simulink model "Nexonar_Test"  (R2018b)
settings: Solver=FixedStepDiscrete  StartTime=0.0  StopTime=7.5  RelTol=1e-3  EnableMultiTasking=on
(part 1 of 2)
settings Model: ExtModeTrigDuration=8  Creator=User  LastModifiedBy=hengw
settings DataIOCC: LimitDataPoints=on  SaveFormat=Array  SaveOutput=off  SaveTime=off
settings OptimizationCC: DefaultUnderspecifiedDataType=single  ExpressionDepthLimit=2147483647  LifeSpan=1  MaxStackSize=512
settings DebuggingCC: UnderspecifiedInitializationDetection=Classic  MergeDetectMultiDrivingBlocksExec=none  SolverPrmCheckMsg=warning  StateNameClashWarn=warning  SFUnexpectedBacktrackingDiag=warning  SFNoUnconditionalDefaultTransitionDiag=warning  SFExecutionAtInitializationDiag=none
settings HardwareCC: ProdBitPerChar=16  ProdBitPerInt=16  ProdBitPerPointer=32  ProdBitPerSizeT=32  ProdBitPerPtrDiffT=32  ProdLargestAtomicInteger=Integer  ProdLargestAtomicFloat=None  ProdWordSize=16  ProdLongLongMode=on  ProdHWDeviceType=Texas Instruments->C2000  TargetBitPerChar=16  TargetBitPerInt=16  TargetLargestAtomicInteger=Integer  TargetIntDivRoundTo=Zero  TargetEndianess=LittleEndian  TargetWordSize=16  TargetHWDeviceType=Texas Instruments->C2000  ProdEqTarget=off
settings ModelReferenceCC: PropagateSignalLabelsOutOfModel=off
settings SFSimCC: SimCustomSourceCode="#include \"i2c_reset.c\""  SimCustomHeaderCode="#include \"i2c_reset.h\""  SimUseLocalCustomCode=off  MATLABDynamicMemAlloc=off
settings RTWCC: SystemTargetFile=ert.tlc  HardwareBoard=TI Delfino F2833x  TemplateMakefile=ert_default_tmf  RTWUseLocalCustomCode=off  RTWUseSimCustomCode=on  CustomSourceCode="#include \"i2c_reset.c\""  CustomHeaderCode="#include \"i2c_reset.h\""  Toolchain=Texas Instruments Code Composer Studio (C2000)
settings CodeAppCC: IgnoreCustomStorageClasses=off  CustomSymbolStrType=$N$R$M  StateflowObjectComments=on  InternalIdentifier=Classic
settings ERTTargetCC: CodeReplacementLibrary=TI C28x  MultiwordLength=2048  ParMdlRefBuildCompliant=off  CPPClassGenCompliant=off  ConvertIfToSwitch=off  SuppressUnreachableDefaultCases=off
settings ConfigComp: CovMetricSettings=dw  CovHtmlReporting=on  CovSaveCumulativeToWorkspaceVar=on  CovSaveSingleToWorkspaceVar=on  CovExternalEMLEnable=off

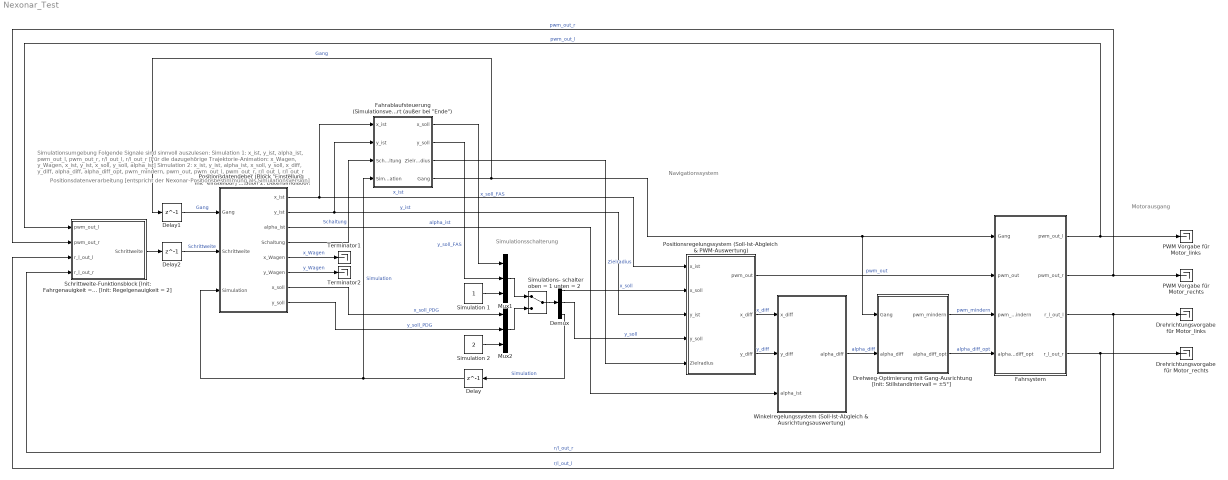
== system Nexonar_Test ==
  note: Simulationsschalterung
  note: Simulationsumgebung
      |
      |
      |
      |
      |
      |
      |
      |
      |
      |
      |
      |
      |
      |
      |
      |
      |
      |
      |
      |
      |
      |
      |
      |
      |
      |
      |
      |
      | Folgende Signale sind sinnvoll auszulesen:
      | Simulation 1: x_ist, y_ist, alpha_ist, pwm_out_l, pwm_out_r, r/l_out_l, r/l_out_r
      | [Für die dazugehörige Trajektorie-Animation: x_Wagen, y_Wagen, x_ist, y_ist, x_soll, y_soll, alpha_ist]
      | Simulation 2: x_ist, y_ist, alpha_ist, x_soll, y_soll, x_diff, y_diff, alpha_diff, alpha_diff_opt, pwm_mindern, pwm_out, pwm_out_l, pwm_out_r, r/l_out_l, r/l_out_r
  note: Navigationssystem
  note: Motorausgang
  note: Positionsdatenverarbeitung
      |
      |
      |
      |
      |
      |
      |
      |
      |
      |
      |
      |
      |
      |
      |
      |
      |
      |
      | [entspricht der Nexonar-Positionsbestimmung
      | als Simulationsversion]
  Delay : Delay  DelayLength=1  InitialCondition=0
  Delay1 : Delay  DelayLength=1  InitialCondition=0
  Delay2 : Delay  DelayLength=1  InitialCondition=0
  Demux : Demux  Outputs=3
  Drehrichtungsvorgabe für Motor_links : Terminator
  Drehrichtungsvorgabe für Motor_rechts : Terminator
  Drehweg-Optimierung mit Gang-Ausrichtung [Init: Stillstandintervall = ±5°] : Stateflow chart  TreatAsAtomicUnit=on
  "Fahrablaufsteuerung (Simulationsversion) [Init: Zielradius = 5mm] Gang = 0: vorwaerts Gang = 1: rueckwaerts Folgende Werte fuer den Ablauf sind einstellbar: - Zielkoordinatenwerte - Gangwert (außer bei \"Ende\")" : Stateflow chart  TreatAsAtomicUnit=on
  Fahrsystem : Stateflow chart  TreatAsAtomicUnit=on
  Mux1 : Mux  Inputs=3
  Mux2 : Mux  Inputs=3
  PWM Vorgabe für Motor_links : Terminator
  PWM Vorgabe für Motor_rechts : Terminator
  "Positionsdatengeber [Block \"Einstellung_Init\" einstellbar] Simulation 1: Fahrsimulation Simulation 2: Datensimulation" : Stateflow chart  TreatAsAtomicUnit=on
  Positionsregelungssystem (Soll-Ist-Abgleich & PWM-Auswertung) : Subsystem
  Schrittweite-Funktionsblock [Init: Fahrgenauigkeit = 10] [Init: Drehgenauigkeit = 30] [Init: Regelgenauigkeit = 2] : MATLAB Function  TreatAsAtomicUnit=on
  Simulation 1 : Constant
  Simulation 2 : Constant  Value=2
  Simulations- schalter oben = 1 unten = 2 : ManualSwitch
  Terminator1 : Terminator
  Terminator2 : Terminator
  Winkelregelungssystem (Soll-Ist-Abgleich & Ausrichtungsauswertung) : Subsystem
  wires:
  "Positionsdatengeber [Block \"Einstellung_Init\" einstellbar] Simulation 1: Fahrsimulation Simulation 2: Datensimulation"/2(y_ist) -> "Fahrablaufsteuerung (Simulationsversion) [Init: Zielradius = 5mm] Gang = 0: vorwaerts Gang = 1: rueckwaerts Folgende Werte fuer den Ablauf sind einstellbar: - Zielkoordinatenwerte - Gangwert (außer bei \"Ende\")"/2(y_ist), Positionsregelungssystem (Soll-Ist-Abgleich & PWM-Auswertung)/3(y_ist)  "y_ist"
  "Fahrablaufsteuerung (Simulationsversion) [Init: Zielradius = 5mm] Gang = 0: vorwaerts Gang = 1: rueckwaerts Folgende Werte fuer den Ablauf sind einstellbar: - Zielkoordinatenwerte - Gangwert (außer bei \"Ende\")"/4(Gang) -> Drehweg-Optimierung mit Gang-Ausrichtung [Init: Stillstandintervall = ±5°]/1(Gang), Fahrsystem/1(Gang), Delay1/1  "Gang"
  Fahrsystem/4(r_l_out_r) -> Schrittweite-Funktionsblock [Init: Fahrgenauigkeit = 10] [Init: Drehgenauigkeit = 30] [Init: Regelgenauigkeit = 2]/4(r_l_out_r), Drehrichtungsvorgabe für Motor_rechts/1  "r/l_out_r"
  Fahrsystem/3(r_l_out_l) -> Drehrichtungsvorgabe für Motor_links/1, Schrittweite-Funktionsblock [Init: Fahrgenauigkeit = 10] [Init: Drehgenauigkeit = 30] [Init: Regelgenauigkeit = 2]/3(r_l_out_l)  "r/l_out_l"
  "Positionsdatengeber [Block \"Einstellung_Init\" einstellbar] Simulation 1: Fahrsimulation Simulation 2: Datensimulation"/1(x_ist) -> "Fahrablaufsteuerung (Simulationsversion) [Init: Zielradius = 5mm] Gang = 0: vorwaerts Gang = 1: rueckwaerts Folgende Werte fuer den Ablauf sind einstellbar: - Zielkoordinatenwerte - Gangwert (außer bei \"Ende\")"/1(x_ist), Positionsregelungssystem (Soll-Ist-Abgleich & PWM-Auswertung)/1(x_ist)  "x_ist"
  Demux/1 -> Positionsregelungssystem (Soll-Ist-Abgleich & PWM-Auswertung)/2(x_soll)  "x_soll"
  Demux/2 -> Positionsregelungssystem (Soll-Ist-Abgleich & PWM-Auswertung)/4(y_soll)  "y_soll"
  Schrittweite-Funktionsblock [Init: Fahrgenauigkeit = 10] [Init: Drehgenauigkeit = 30] [Init: Regelgenauigkeit = 2]/1(Schrittweite) -> Delay2/1
  Fahrsystem/1(pwm_out_l) -> PWM Vorgabe für Motor_links/1, Schrittweite-Funktionsblock [Init: Fahrgenauigkeit = 10] [Init: Drehgenauigkeit = 30] [Init: Regelgenauigkeit = 2]/1(pwm_out_l)  "pwm_out_l"
  Fahrsystem/2(pwm_out_r) -> PWM Vorgabe für Motor_rechts/1, Schrittweite-Funktionsblock [Init: Fahrgenauigkeit = 10] [Init: Drehgenauigkeit = 30] [Init: Regelgenauigkeit = 2]/2(pwm_out_r)  "pwm_out_r"
  Delay1/1 -> "Positionsdatengeber [Block \"Einstellung_Init\" einstellbar] Simulation 1: Fahrsimulation Simulation 2: Datensimulation"/1(Gang)  "Gang"
  Positionsregelungssystem (Soll-Ist-Abgleich & PWM-Auswertung)/1(pwm_out) -> Fahrsystem/2(pwm_out)  "pwm_out"
  Positionsregelungssystem (Soll-Ist-Abgleich & PWM-Auswertung)/3(y_diff) -> Winkelregelungssystem (Soll-Ist-Abgleich & Ausrichtungsauswertung)/2(y_diff)  "y_diff"
  Winkelregelungssystem (Soll-Ist-Abgleich & Ausrichtungsauswertung)/1(alpha_diff) -> Drehweg-Optimierung mit Gang-Ausrichtung [Init: Stillstandintervall = ±5°]/2(alpha_diff)  "alpha_diff"
  Drehweg-Optimierung mit Gang-Ausrichtung [Init: Stillstandintervall = ±5°]/2(alpha_diff_opt) -> Fahrsystem/4(alpha_diff_opt)  "alpha_diff_opt"
  Positionsregelungssystem (Soll-Ist-Abgleich & PWM-Auswertung)/2(x_diff) -> Winkelregelungssystem (Soll-Ist-Abgleich & Ausrichtungsauswertung)/1(x_diff)  "x_diff"
  "Positionsdatengeber [Block \"Einstellung_Init\" einstellbar] Simulation 1: Fahrsimulation Simulation 2: Datensimulation"/3(alpha_ist) -> Winkelregelungssystem (Soll-Ist-Abgleich & Ausrichtungsauswertung)/3(alpha_ist)  "alpha_ist"
  Simulation 1/1 -> Mux1/3
  Simulation 2/1 -> Mux2/3
  Demux/3 -> Delay/1  "Simulation"
  "Positionsdatengeber [Block \"Einstellung_Init\" einstellbar] Simulation 1: Fahrsimulation Simulation 2: Datensimulation"/8(y_soll) -> Mux2/2  "y_soll_PDG"
  "Positionsdatengeber [Block \"Einstellung_Init\" einstellbar] Simulation 1: Fahrsimulation Simulation 2: Datensimulation"/7(x_soll) -> Mux2/1  "x_soll_PDG"
  "Fahrablaufsteuerung (Simulationsversion) [Init: Zielradius = 5mm] Gang = 0: vorwaerts Gang = 1: rueckwaerts Folgende Werte fuer den Ablauf sind einstellbar: - Zielkoordinatenwerte - Gangwert (außer bei \"Ende\")"/2(y_soll) -> Mux1/2  "y_soll_FAS"
  "Fahrablaufsteuerung (Simulationsversion) [Init: Zielradius = 5mm] Gang = 0: vorwaerts Gang = 1: rueckwaerts Folgende Werte fuer den Ablauf sind einstellbar: - Zielkoordinatenwerte - Gangwert (außer bei \"Ende\")"/1(x_soll) -> Mux1/1  "x_soll_FAS"
  Delay2/1 -> "Positionsdatengeber [Block \"Einstellung_Init\" einstellbar] Simulation 1: Fahrsimulation Simulation 2: Datensimulation"/2(Schrittweite)  "Schrittweite"
  "Positionsdatengeber [Block \"Einstellung_Init\" einstellbar] Simulation 1: Fahrsimulation Simulation 2: Datensimulation"/4(Schaltung) -> "Fahrablaufsteuerung (Simulationsversion) [Init: Zielradius = 5mm] Gang = 0: vorwaerts Gang = 1: rueckwaerts Folgende Werte fuer den Ablauf sind einstellbar: - Zielkoordinatenwerte - Gangwert (außer bei \"Ende\")"/3(Schaltung)  "Schaltung"
  "Fahrablaufsteuerung (Simulationsversion) [Init: Zielradius = 5mm] Gang = 0: vorwaerts Gang = 1: rueckwaerts Folgende Werte fuer den Ablauf sind einstellbar: - Zielkoordinatenwerte - Gangwert (außer bei \"Ende\")"/3(Zielradius) -> Positionsregelungssystem (Soll-Ist-Abgleich & PWM-Auswertung)/5(Zielradius)  "Zielradius"
  Simulations- schalter oben = 1 unten = 2/1 -> Demux/1
  Mux2/1 -> Simulations- schalter oben = 1 unten = 2/2
  Mux1/1 -> Simulations- schalter oben = 1 unten = 2/1
  Delay/1 -> "Positionsdatengeber [Block \"Einstellung_Init\" einstellbar] Simulation 1: Fahrsimulation Simulation 2: Datensimulation"/3(Simulation), "Fahrablaufsteuerung (Simulationsversion) [Init: Zielradius = 5mm] Gang = 0: vorwaerts Gang = 1: rueckwaerts Folgende Werte fuer den Ablauf sind einstellbar: - Zielkoordinatenwerte - Gangwert (außer bei \"Ende\")"/4(Simulation)  "Simulation"
  Drehweg-Optimierung mit Gang-Ausrichtung [Init: Stillstandintervall = ±5°]/1(pwm_mindern) -> Fahrsystem/3(pwm_mindern)  "pwm_mindern"
  "Positionsdatengeber [Block \"Einstellung_Init\" einstellbar] Simulation 1: Fahrsimulation Simulation 2: Datensimulation"/5(x_Wagen) -> Terminator1/1  "x_Wagen"
  "Positionsdatengeber [Block \"Einstellung_Init\" einstellbar] Simulation 1: Fahrsimulation Simulation 2: Datensimulation"/6(y_Wagen) -> Terminator2/1  "y_Wagen"

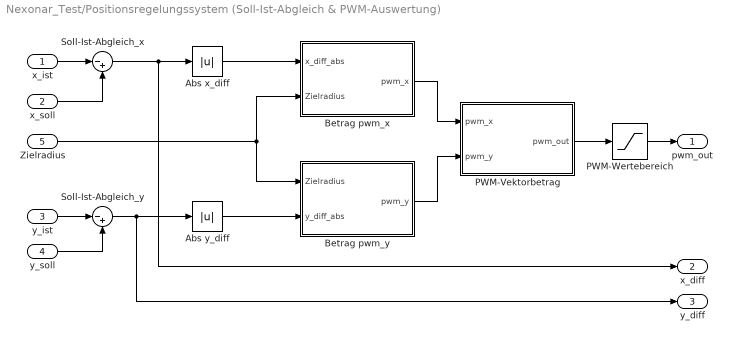
== system Nexonar_Test/Positionsregelungssystem (Soll-Ist-Abgleich & PWM-Auswertung) ==
  x_ist : Inport
  x_soll : Inport  Port=2
  y_ist : Inport  Port=3
  y_soll : Inport  Port=4
  Zielradius : Inport  Port=5
  Abs x_diff : Abs  SampleTime=0.01
  Abs y_diff : Abs  SampleTime=0.01
  Betrag pwm_x : MATLAB Function  TreatAsAtomicUnit=on  SystemSampleTime=0.01
  Betrag pwm_y : MATLAB Function  TreatAsAtomicUnit=on  SystemSampleTime=0.01
  PWM-Vektorbetrag : MATLAB Function  TreatAsAtomicUnit=on
  PWM-Wertebereich : Saturate  UpperLimit=100  LowerLimit=0
  Soll-Ist-Abgleich_x : Sum  Inputs=|-+  SampleTime=0.01
  Soll-Ist-Abgleich_y : Sum  Inputs=|-+  AccumDataTypeStr=double  SampleTime=0.01
  pwm_out : Outport
  x_diff : Outport  Port=2
  y_diff : Outport  Port=3
  wires:
  Soll-Ist-Abgleich_x/1 -> x_diff/1, Abs x_diff/1
  Abs x_diff/1 -> Betrag pwm_x/1(x_diff_abs)
  x_soll/1 -> Soll-Ist-Abgleich_x/2
  x_ist/1 -> Soll-Ist-Abgleich_x/1
  y_ist/1 -> Soll-Ist-Abgleich_y/1
  y_soll/1 -> Soll-Ist-Abgleich_y/2
  Soll-Ist-Abgleich_y/1 -> Abs y_diff/1, y_diff/1
  Abs y_diff/1 -> Betrag pwm_y/2(y_diff_abs)
  PWM-Wertebereich/1 -> pwm_out/1
  PWM-Vektorbetrag/1(pwm_out) -> PWM-Wertebereich/1
  Betrag pwm_x/1(pwm_x) -> PWM-Vektorbetrag/1(pwm_x)
  Betrag pwm_y/1(pwm_y) -> PWM-Vektorbetrag/2(pwm_y)
  Zielradius/1 -> Betrag pwm_y/1(Zielradius), Betrag pwm_x/2(Zielradius)

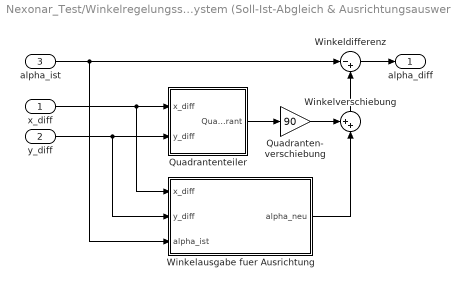
== system Nexonar_Test/Winkelregelungssystem (Soll-Ist-Abgleich & Ausrichtungsauswertung) ==
  x_diff : Inport
  y_diff : Inport  Port=2
  alpha_ist : Inport  Port=3
  Quadranten- verschiebung : Gain  Gain=90
  Quadrantenteiler : Stateflow chart  TreatAsAtomicUnit=on
  Winkelausgabe fuer Ausrichtung : Stateflow chart  TreatAsAtomicUnit=on
  Winkeldifferenz : Sum  Inputs=|-+
  Winkelverschiebung : Sum  Inputs=++|
  alpha_diff : Outport
  wires:
  alpha_ist/1 -> Winkelausgabe fuer Ausrichtung/3(alpha_ist), Winkeldifferenz/1
  y_diff/1 -> Winkelausgabe fuer Ausrichtung/2(y_diff), Quadrantenteiler/2(y_diff)
  Winkelausgabe fuer Ausrichtung/1(alpha_neu) -> Winkelverschiebung/2
  Winkelverschiebung/1 -> Winkeldifferenz/2
  x_diff/1 -> Winkelausgabe fuer Ausrichtung/1(x_diff), Quadrantenteiler/1(x_diff)
  Quadrantenteiler/1(Quadrant) -> Quadranten- verschiebung/1
  Winkeldifferenz/1 -> alpha_diff/1
  Quadranten- verschiebung/1 -> Winkelverschiebung/1

== stateflow chart Nexonar_Test/Fahrablaufsteuerung (Simulationsversion) [Init: Zielradius = 5mm] Gang = 0: vorwaerts Gang = 1: rueckwaerts Folgende Werte fuer den Ablauf sind einstellbar: - Zielkoordinatenwerte - Gangwert (außer bei "Ende") ==
  state Parken3 [commented out]
    entry:
    x_soll = 1700;
    y_soll = -100;
  state Uebergabe3 [commented out]
    state Uebergabepunkt_x_Richtung [commented out]
      entry:
      x_soll = 1325;
      y_soll = y_least;
    state Wechsel_1 [commented out]
      entry:
      Counter = Counter + 1;
    state Uebergabepunkt_y_Richtung [commented out]
      entry:
      x_soll = x_least;
      y_soll = 100;
    state Warten_Uebergabe [commented out]
    state Wechsel_2 [commented out]
      entry:
      Counter = Counter + 1;
    (default) -> Uebergabe3.Uebergabepunkt_x_Richtung [commented out] : {Counter = 0}
    Uebergabe3.Uebergabepunkt_x_Richtung -> Uebergabe3.Wechsel_1 [commented out] : [abs(x_soll - x_ist) <= Zielradius && abs(y_soll - y_ist) <= Zielradius]
        | {x_least = x_soll; y_least = y_soll;}
    Uebergabe3.Wechsel_1 -> Uebergabe3.Uebergabepunkt_y_Richtung [commented out]
    Uebergabe3.Uebergabepunkt_y_Richtung -> Uebergabe3.Warten_Uebergabe [commented out] : [abs(x_soll - x_ist) <= Zielradius && abs(y_soll - y_ist) <= Zielradius]
    Uebergabe3.Warten_Uebergabe -> Uebergabe3.Wechsel_2 [commented out] : [after(1,sec)]
  state Sammeln3 [commented out]
    state Anfahrpunkt_1 [commented out]
      entry:
      x_soll = 1450;
      y_soll = 0;
    state Wechsel_1 [commented out]
      entry:
      Counter = Counter + 1;
    state Anfahrpunkt_2 [commented out]
      entry:
      x_soll = 1200;
      y_soll = 25;
    state Wechsel_2 [commented out]
      entry:
      Counter = Counter + 1;
    state Anfahrpunkt_3 [commented out]
      entry:
      x_soll = 800;
      y_soll = 400;
    state Wechsel_3 [commented out]
      entry:
      Counter = Counter + 1;
    state Anfahrpunkt_4 [commented out]
      entry:
      x_soll = 900;
      y_soll = 650;
    state Wechsel_4 [commented out]
      entry:
      Counter = Counter + 1;
    state Anfahrpunkt_5 [commented out]
      entry:
      x_soll = 750;
      y_soll = 850;
    state Wechsel_5 [commented out]
      entry:
      Counter = Counter + 1;
    state Anfahrpunkt_6 [commented out]
      entry:
      x_soll = 600;
      y_soll = 850;
    state Wechsel_6 [commented out]
      entry:
      Counter = Counter + 1;
    state Anfahrpunkt_7 [commented out]
      entry:
      x_soll = 500;
      y_soll = 850;
    state Wechsel_7 [commented out]
      entry:
      Counter = Counter + 1;
    state Anfahrpunkt_8 [commented out]
      entry:
      x_soll = 200;
      y_soll = 750;
    state Wechsel_8 [commented out]
      entry:
      Counter = Counter + 1;
    state Anfahrpunkt_9 [commented out]
      entry:
      x_soll = 400;
      y_soll = 50;
    state Wechsel_9 [commented out]
      entry:
      Counter = Counter + 1;
    state Anfahrpunkt_10 [commented out]
      entry:
      x_soll = 1200;
      y_soll = 50;
    state Wechsel_10 [commented out]
      entry:
      Counter = Counter + 1;
    state Anfahrpunkt_11 [commented out]
      entry:
      x_soll = 1350;
      y_soll = -100;
    state Wechsel_11 [commented out]
      entry:
      Counter = Counter + 1;
    (default) -> Sammeln3.Anfahrpunkt_1 [commented out] : {Counter = 0}
    Sammeln3.Anfahrpunkt_1 -> Sammeln3.Wechsel_1 [commented out] : [abs(x_soll - x_ist) <= Zielradius && abs(y_soll - y_ist) <= Zielradius]
    Sammeln3.Wechsel_1 -> Sammeln3.Anfahrpunkt_2 [commented out]
    Sammeln3.Anfahrpunkt_2 -> Sammeln3.Wechsel_2 [commented out] : [abs(x_soll - x_ist) <= Zielradius && abs(y_soll - y_ist) <= Zielradius]
    Sammeln3.Wechsel_2 -> Sammeln3.Anfahrpunkt_3 [commented out]
    Sammeln3.Anfahrpunkt_3 -> Sammeln3.Wechsel_3 [commented out] : [abs(x_soll - x_ist) <= Zielradius && abs(y_soll - y_ist) <= Zielradius]
    Sammeln3.Wechsel_3 -> Sammeln3.Anfahrpunkt_4 [commented out]
    Sammeln3.Anfahrpunkt_4 -> Sammeln3.Wechsel_4 [commented out] : [abs(x_soll - x_ist) <= Zielradius && abs(y_soll - y_ist) <= Zielradius]
    Sammeln3.Wechsel_4 -> Sammeln3.Anfahrpunkt_5 [commented out]
    Sammeln3.Anfahrpunkt_5 -> Sammeln3.Wechsel_5 [commented out] : [abs(x_soll - x_ist) <= Zielradius && abs(y_soll - y_ist) <= Zielradius]
    Sammeln3.Wechsel_5 -> Sammeln3.Anfahrpunkt_6 [commented out]
    Sammeln3.Anfahrpunkt_6 -> Sammeln3.Wechsel_6 [commented out] : [abs(x_soll - x_ist) <= Zielradius && abs(y_soll - y_ist) <= Zielradius]
    Sammeln3.Wechsel_6 -> Sammeln3.Anfahrpunkt_7 [commented out]
    Sammeln3.Anfahrpunkt_7 -> Sammeln3.Wechsel_7 [commented out] : [abs(x_soll - x_ist) <= Zielradius && abs(y_soll - y_ist) <= Zielradius]
    Sammeln3.Wechsel_7 -> Sammeln3.Anfahrpunkt_8 [commented out]
    Sammeln3.Anfahrpunkt_8 -> Sammeln3.Wechsel_8 [commented out] : [abs(x_soll - x_ist) <= Zielradius && abs(y_soll - y_ist) <= Zielradius]
    Sammeln3.Wechsel_8 -> Sammeln3.Anfahrpunkt_9 [commented out]
    Sammeln3.Anfahrpunkt_9 -> Sammeln3.Wechsel_9 [commented out] : [abs(x_soll - x_ist) <= Zielradius && abs(y_soll - y_ist) <= Zielradius]
    Sammeln3.Wechsel_9 -> Sammeln3.Anfahrpunkt_10 [commented out]
    Sammeln3.Anfahrpunkt_10 -> Sammeln3.Wechsel_10 [commented out] : [abs(x_soll - x_ist) <= Zielradius && abs(y_soll - y_ist) <= Zielradius]
    Sammeln3.Wechsel_10 -> Sammeln3.Anfahrpunkt_11 [commented out]
    Sammeln3.Anfahrpunkt_11 -> Sammeln3.Wechsel_11 [commented out] : [abs(x_soll - x_ist) <= Zielradius && abs(y_soll - y_ist) <= Zielradius]
  state Parken2 [commented out]
    entry:
    x_soll = 1700;
    y_soll = -150;
  state Uebergabe2 [commented out]
    state Uebergabepunkt_x_Richtung [commented out]
      entry:
      x_soll = 1325;
      y_soll = y_least;
    state Wechsel_1 [commented out]
      entry:
      Counter = Counter + 1;
    state Uebergabepunkt_y_Richtung [commented out]
      entry:
      x_soll = x_least;
      y_soll = 100;
    state Warten_Uebergabe [commented out]
    state Wechsel_2 [commented out]
      entry:
      Counter = Counter + 1;
    (default) -> Uebergabe2.Uebergabepunkt_x_Richtung [commented out] : {Counter = 0}
    Uebergabe2.Uebergabepunkt_x_Richtung -> Uebergabe2.Wechsel_1 [commented out] : [abs(x_soll - x_ist) <= Zielradius && abs(y_soll - y_ist) <= Zielradius]
        | {x_least = x_soll; y_least = y_soll;}
    Uebergabe2.Wechsel_1 -> Uebergabe2.Uebergabepunkt_y_Richtung [commented out]
    Uebergabe2.Uebergabepunkt_y_Richtung -> Uebergabe2.Warten_Uebergabe [commented out] : [abs(x_soll - x_ist) <= Zielradius && abs(y_soll - y_ist) <= Zielradius]
    Uebergabe2.Warten_Uebergabe -> Uebergabe2.Wechsel_2 [commented out] : [after(1,sec)]
  state Sammeln2 [commented out]
    state Anfahrpunkt_1 [commented out]
      entry:
      x_soll = 1400;
      y_soll = 50;
    state Wechsel_1 [commented out]
      entry:
      Counter = Counter + 1;
    state Anfahrpunkt_2 [commented out]
      entry:
      x_soll = 550;
      y_soll = 50;
    state Wechsel_2 [commented out]
      entry:
      Counter = Counter + 1;
    state Anfahrpunkt_3 [commented out]
      entry:
      x_soll = 975;
      y_soll = 600;
    state Wechsel_3 [commented out]
      entry:
      Counter = Counter + 1;
    state Anfahrpunkt_4 [commented out]
      entry:
      x_soll = 925;
      y_soll = 750;
    state Wechsel_4 [commented out]
      entry:
      Counter = Counter + 1;
    state Anfahrpunkt_5 [commented out]
      entry:
      x_soll = 850;
      y_soll = 800;
    state Wechsel_5 [commented out]
      entry:
      Counter = Counter + 1;
    state Anfahrpunkt_6 [commented out]
      entry:
      x_soll = 750;
      y_soll = 850;
    state Wechsel_6 [commented out]
      entry:
      Counter = Counter + 1;
    state Anfahrpunkt_7 [commented out]
      entry:
      x_soll = 600;
      y_soll = 875;
    state Wechsel_7 [commented out]
      entry:
      Counter = Counter + 1;
    state Anfahrpunkt_8 [commented out]
      entry:
      x_soll = 500;
      y_soll = 875;
    state Wechsel_8 [commented out]
      entry:
      Counter = Counter + 1;
    state Anfahrpunkt_9 [commented out]
      entry:
      x_soll = 350;
      y_soll = 850;
    state Wechsel_9 [commented out]
      entry:
      Counter = Counter + 1;
    state Anfahrpunkt_10 [commented out]
      entry:
      x_soll = 250;
      y_soll = 800;
    state Wechsel_10 [commented out]
      entry:
      Counter = Counter + 1;
    state Anfahrpunkt_11 [commented out]
      entry:
      x_soll = 175;
      y_soll = 750;
    state Wechsel_11 [commented out]
      entry:
      Counter = Counter + 1;
    state Anfahrpunkt_12 [commented out]
      entry:
      x_soll = 125;
      y_soll = 600;
    state Wechsel_12 [commented out]
      entry:
      Counter = Counter + 1;
    state Anfahrpunkt_13 [commented out]
      entry:
      x_soll = 400;
      y_soll = 50;
    state Wechsel_13 [commented out]
      entry:
      Counter = Counter + 1;
    state Anfahrpunkt_14 [commented out]
      entry:
      x_soll = 1200;
      y_soll = 50;
    state Wechsel_14 [commented out]
      entry:
      Counter = Counter + 1;
    state Anfahrpunkt_15 [commented out]
      entry:
      x_soll = 1350;
      y_soll = -150;
    state Wechsel_15 [commented out]
      entry:
      Counter = Counter + 1;
    (default) -> Sammeln2.Anfahrpunkt_1 [commented out] : {Counter = 0}
    Sammeln2.Anfahrpunkt_1 -> Sammeln2.Wechsel_1 [commented out] : [abs(x_soll - x_ist) <= Zielradius && abs(y_soll - y_ist) <= Zielradius]
    Sammeln2.Wechsel_1 -> Sammeln2.Anfahrpunkt_2 [commented out]
    Sammeln2.Anfahrpunkt_2 -> Sammeln2.Wechsel_2 [commented out] : [abs(x_soll - x_ist) <= Zielradius && abs(y_soll - y_ist) <= Zielradius]
    Sammeln2.Wechsel_2 -> Sammeln2.Anfahrpunkt_3 [commented out]
    Sammeln2.Anfahrpunkt_3 -> Sammeln2.Wechsel_3 [commented out] : [abs(x_soll - x_ist) <= Zielradius && abs(y_soll - y_ist) <= Zielradius]
    Sammeln2.Wechsel_3 -> Sammeln2.Anfahrpunkt_4 [commented out]
    Sammeln2.Anfahrpunkt_4 -> Sammeln2.Wechsel_4 [commented out] : [abs(x_soll - x_ist) <= Zielradius && abs(y_soll - y_ist) <= Zielradius]
    Sammeln2.Wechsel_4 -> Sammeln2.Anfahrpunkt_5 [commented out]
    Sammeln2.Anfahrpunkt_5 -> Sammeln2.Wechsel_5 [commented out] : [abs(x_soll - x_ist) <= Zielradius && abs(y_soll - y_ist) <= Zielradius]
    Sammeln2.Wechsel_5 -> Sammeln2.Anfahrpunkt_6 [commented out]
    Sammeln2.Anfahrpunkt_6 -> Sammeln2.Wechsel_6 [commented out] : [abs(x_soll - x_ist) <= Zielradius && abs(y_soll - y_ist) <= Zielradius]
    Sammeln2.Wechsel_6 -> Sammeln2.Anfahrpunkt_7 [commented out]
    Sammeln2.Anfahrpunkt_7 -> Sammeln2.Wechsel_7 [commented out] : [abs(x_soll - x_ist) <= Zielradius && abs(y_soll - y_ist) <= Zielradius]
    Sammeln2.Wechsel_7 -> Sammeln2.Anfahrpunkt_8 [commented out]
    Sammeln2.Anfahrpunkt_8 -> Sammeln2.Wechsel_8 [commented out] : [abs(x_soll - x_ist) <= Zielradius && abs(y_soll - y_ist) <= Zielradius]
    Sammeln2.Wechsel_8 -> Sammeln2.Anfahrpunkt_9 [commented out]
    Sammeln2.Anfahrpunkt_9 -> Sammeln2.Wechsel_9 [commented out] : [abs(x_soll - x_ist) <= Zielradius && abs(y_soll - y_ist) <= Zielradius]
    Sammeln2.Wechsel_9 -> Sammeln2.Anfahrpunkt_10 [commented out]
    Sammeln2.Anfahrpunkt_10 -> Sammeln2.Wechsel_10 [commented out] : [abs(x_soll - x_ist) <= Zielradius && abs(y_soll - y_ist) <= Zielradius]
    Sammeln2.Wechsel_10 -> Sammeln2.Anfahrpunkt_11 [commented out]
    Sammeln2.Anfahrpunkt_11 -> Sammeln2.Wechsel_11 [commented out] : [abs(x_soll - x_ist) <= Zielradius && abs(y_soll - y_ist) <= Zielradius]
    Sammeln2.Wechsel_11 -> Sammeln2.Anfahrpunkt_12 [commented out]
    Sammeln2.Anfahrpunkt_12 -> Sammeln2.Wechsel_12 [commented out] : [abs(x_soll - x_ist) <= Zielradius && abs(y_soll - y_ist) <= Zielradius]
    Sammeln2.Wechsel_12 -> Sammeln2.Anfahrpunkt_13 [commented out]
    Sammeln2.Anfahrpunkt_13 -> Sammeln2.Wechsel_13 [commented out] : [abs(x_soll - x_ist) <= Zielradius && abs(y_soll - y_ist) <= Zielradius]
    Sammeln2.Wechsel_13 -> Anfahrpunkt_14 [commented out]
    Anfahrpunkt_14 -> Wechsel_14 [commented out] : [abs(x_soll - x_ist) <= Zielradius && abs(y_soll - y_ist) <= Zielradius]
    Wechsel_14 -> Anfahrpunkt_15 [commented out]
    Anfahrpunkt_15 -> Wechsel_15 [commented out] : [abs(x_soll - x_ist) <= Zielradius && abs(y_soll - y_ist) <= Zielradius]
  state Parken1 [commented out]
    entry:
    x_soll = 1670;
    y_soll = -150;
  state Uebergabe1 [commented out]
    state Uebergabepunkt_x_Richtung [commented out]
      entry:
      x_soll = 1420;
      y_soll = y_least;
    state Wechsel_1 [commented out]
      entry:
      Counter = Counter + 1;
    state Uebergabepunkt_y_Richtung [commented out]
      entry:
      x_soll = x_least;
      y_soll = 90;
    state Warten_Uebergabe [commented out]
    state Wechsel_2 [commented out]
      entry:
      Counter = Counter + 1;
    (default) -> Uebergabe1.Uebergabepunkt_x_Richtung [commented out] : {Counter = 0}
    Uebergabe1.Uebergabepunkt_x_Richtung -> Uebergabe1.Wechsel_1 [commented out] : [abs(x_soll - x_ist) <= Zielradius && abs(y_soll - y_ist) <= Zielradius]
        | {x_least = x_soll; y_least = y_soll;}
    Uebergabe1.Wechsel_1 -> Uebergabe1.Uebergabepunkt_y_Richtung [commented out]
    Uebergabe1.Uebergabepunkt_y_Richtung -> Uebergabe1.Warten_Uebergabe [commented out] : [abs(x_soll - x_ist) <= Zielradius && abs(y_soll - y_ist) <= Zielradius]
    Uebergabe1.Warten_Uebergabe -> Uebergabe1.Wechsel_2 [commented out] : [after(1,sec)]
  state Sammeln1 [commented out]
    state Anfahrpunkt_1 [commented out]
      entry:
      x_soll = 1500;
      y_soll = 0;
    state Wechsel_1 [commented out]
      entry:
      Counter = Counter + 1;
    state Anfahrpunkt_2 [commented out]
      entry:
      x_soll = 1200;
      y_soll = 100;
    state Wechsel_2 [commented out]
      entry:
      Counter = Counter + 1;
    state Anfahrpunkt_3 [commented out]
      entry:
      x_soll = 1000;
      y_soll = 200;
    state Wechsel_3 [commented out]
      entry:
      Counter = Counter + 1;
    state Anfahrpunkt_4 [commented out]
      entry:
      x_soll = 900;
      y_soll = 400;
    state Wechsel_4 [commented out]
      entry:
      Counter = Counter + 1;
    state Anfahrpunkt_5 [commented out]
      entry:
      x_soll = 950;
      y_soll = 570;
    state Wechsel_5 [commented out]
      entry:
      Counter = Counter + 1;
    state Anfahrpunkt_6 [commented out]
      entry:
      x_soll = 640;
      y_soll = 750;
      Sammeln1.Anfahrpunkt_6 -> Sammeln1.Anfahrpunkt_6 [commented out]
    state Wechsel_6 [commented out]
      entry:
      Counter = Counter + 1;
    state Anfahrpunkt_7 [commented out]
      entry:
      x_soll = 450;
      y_soll = 820;
    state Wechsel_7 [commented out]
      entry:
      Counter = Counter + 1;
    state Anfahrpunkt_8 [commented out]
      entry:
      x_soll = 360;
      y_soll = 720;
    state Wechsel_8 [commented out]
      entry:
      Counter = Counter + 1;
    state Anfahrpunkt_9 [commented out]
      entry:
      x_soll = 370;
      y_soll = 380;
    state Wechsel_9 [commented out]
      entry:
      Counter = Counter + 1;
    state Anfahrpunkt_10 [commented out]
      entry:
      x_soll = 650;
      y_soll = 80;
    state Wechsel_10 [commented out]
      entry:
      Counter = Counter + 1;
    state Anfahrpunkt_11 [commented out]
      entry:
      x_soll = 1100;
      y_soll = 80;
    state Wechsel_11 [commented out]
      entry:
      Counter = Counter + 1;
    state Anfahrpunkt_12 [commented out]
      entry:
      x_soll = 1240;
      y_soll = -30;
    state Wechsel_12 [commented out]
      entry:
      Counter = Counter + 1;
    state Anfahrpunkt_13 [commented out]
      entry:
      x_soll = 1430;
      y_soll = -80;
    state Wechsel_13 [commented out]
      entry:
      Counter = Counter + 1;
    (default) -> Sammeln1.Anfahrpunkt_1 [commented out] : {Counter = 0}
    Sammeln1.Anfahrpunkt_1 -> Sammeln1.Wechsel_1 [commented out] : [abs(x_soll - x_ist) <= Zielradius && abs(y_soll - y_ist) <= Zielradius]
    Sammeln1.Wechsel_1 -> Sammeln1.Anfahrpunkt_2 [commented out]
    Sammeln1.Anfahrpunkt_2 -> Sammeln1.Wechsel_2 [commented out] : [abs(x_soll - x_ist) <= Zielradius && abs(y_soll - y_ist) <= Zielradius]
    Sammeln1.Wechsel_2 -> Sammeln1.Anfahrpunkt_3 [commented out]
    Sammeln1.Anfahrpunkt_3 -> Sammeln1.Wechsel_3 [commented out] : [abs(x_soll - x_ist) <= Zielradius && abs(y_soll - y_ist) <= Zielradius]
    Sammeln1.Wechsel_3 -> Sammeln1.Anfahrpunkt_4 [commented out]
    Sammeln1.Anfahrpunkt_4 -> Sammeln1.Wechsel_4 [commented out] : [abs(x_soll - x_ist) <= Zielradius && abs(y_soll - y_ist) <= Zielradius]
    Sammeln1.Wechsel_4 -> Sammeln1.Anfahrpunkt_5 [commented out]
    Sammeln1.Anfahrpunkt_5 -> Sammeln1.Wechsel_5 [commented out] : [abs(x_soll - x_ist) <= Zielradius && abs(y_soll - y_ist) <= Zielradius]
    Sammeln1.Wechsel_5 -> Sammeln1.Anfahrpunkt_6 [commented out]
    Sammeln1.Anfahrpunkt_6 -> Sammeln1.Wechsel_6 [commented out] : [abs(x_soll - x_ist) <= Zielradius && abs(y_soll - y_ist) <= Zielradius]
    Sammeln1.Wechsel_6 -> Sammeln1.Anfahrpunkt_7 [commented out]
    Sammeln1.Anfahrpunkt_7 -> Sammeln1.Wechsel_7 [commented out] : [abs(x_soll - x_ist) <= Zielradius && abs(y_soll - y_ist) <= Zielradius]
    Sammeln1.Wechsel_7 -> Sammeln1.Anfahrpunkt_8 [commented out]
    Sammeln1.Anfahrpunkt_8 -> Sammeln1.Wechsel_8 [commented out] : [abs(x_soll - x_ist) <= Zielradius && abs(y_soll - y_ist) <= Zielradius]
    Sammeln1.Wechsel_8 -> Sammeln1.Anfahrpunkt_9 [commented out]
    Sammeln1.Anfahrpunkt_9 -> Sammeln1.Wechsel_9 [commented out] : [abs(x_soll - x_ist) <= Zielradius && abs(y_soll - y_ist) <= Zielradius]
    Sammeln1.Wechsel_9 -> Sammeln1.Anfahrpunkt_10 [commented out]
    Sammeln1.Anfahrpunkt_10 -> Sammeln1.Wechsel_10 [commented out] : [abs(x_soll - x_ist) <= Zielradius && abs(y_soll - y_ist) <= Zielradius]
    Sammeln1.Wechsel_10 -> Sammeln1.Anfahrpunkt_11 [commented out]
    Sammeln1.Anfahrpunkt_11 -> Sammeln1.Wechsel_11 [commented out] : [abs(x_soll - x_ist) <= Zielradius && abs(y_soll - y_ist) <= Zielradius]
    Sammeln1.Wechsel_11 -> Sammeln1.Anfahrpunkt_12 [commented out]
    Sammeln1.Anfahrpunkt_12 -> Sammeln1.Wechsel_12 [commented out] : [abs(x_soll - x_ist) <= Zielradius && abs(y_soll - y_ist) <= Zielradius]
    Sammeln1.Wechsel_12 -> Sammeln1.Anfahrpunkt_13 [commented out]
    Sammeln1.Anfahrpunkt_13 -> Sammeln1.Wechsel_13 [commented out] : [abs(x_soll - x_ist) <= Zielradius && abs(y_soll - y_ist) <= Zielradius]
  state Start_Einstellung_Init
    entry:
    Zielradius = 10;
  state Parken
    state Parken_1
      entry:
      x_soll = 1440;
      y_soll = -50;
    state Wechsel_1
      entry:
      Counter = Counter + 1;
    state Parken_2
      entry:
      x_soll = 1650;
      y_soll = -150;
    state Wechsel_2
      entry:
      Counter = Counter + 1;
    state Parken_3
      entry:
      x_soll = 1675;
      y_soll = -152;
    state Wechsel_3
      entry:
      Counter = Counter + 1;
    (default) -> Parken_1 : {Counter = 0}
    Parken_1 -> Parken.Wechsel_1 : [abs(x_soll - x_ist) <= Zielradius && abs(y_soll - y_ist) <= Zielradius]
    Parken.Wechsel_1 -> Parken_2
    Parken_2 -> Parken.Wechsel_2 : [abs(x_soll - x_ist) <= Zielradius && abs(y_soll - y_ist) <= Zielradius]
    Parken.Wechsel_2 -> Parken_3
    Parken_3 -> Parken.Wechsel_3 : [abs(x_soll - x_ist) <= Zielradius && abs(y_soll - y_ist) <= Zielradius]
  state Uebergabe
    state Uebergabepunkt_x_Richtung
      entry:
      x_soll = 1420;
      y_soll = y_least;
    state Wechsel_1
      entry:
      Counter = Counter + 1;
    state Uebergabepunkt_y_Richtung
      entry:
      x_soll = x_least;
      y_soll = 5;
    state Warten_Uebergabe
    state Wechsel_2
      entry:
      Counter = Counter + 1;
    (default) -> Uebergabe.Uebergabepunkt_x_Richtung : {Counter = 0}
    Uebergabe.Uebergabepunkt_x_Richtung -> Uebergabe.Wechsel_1 : [abs(x_soll - x_ist) <= Zielradius && abs(y_soll - y_ist) <= Zielradius]
        | {x_least = x_soll; y_least = y_soll;}
    Uebergabe.Wechsel_1 -> Uebergabe.Uebergabepunkt_y_Richtung
    Uebergabe.Uebergabepunkt_y_Richtung -> Uebergabe.Warten_Uebergabe : [abs(x_soll - x_ist) <= Zielradius && abs(y_soll - y_ist) <= Zielradius]
    Uebergabe.Warten_Uebergabe -> Uebergabe.Wechsel_2 : [after(1,sec)]
  state Sammeln
    state Anfahrpunkt_1
      entry:
      x_soll = 1560;
      y_soll = 40;
    state Wechsel_1
      entry:
      Counter = Counter + 1;
    state Anfahrpunkt_2
      entry:
      x_soll = 1200;
      y_soll = 40;
    state Wechsel_2
      entry:
      Counter = Counter + 1;
    state Anfahrpunkt_3
      entry:
      x_soll = 800;
      y_soll = 400;
    state Wechsel_3
      entry:
      Counter = Counter + 1;
    state Anfahrpunkt_4
      entry:
      x_soll = 975;
      y_soll = 650;
    state Wechsel_4
      entry:
      Counter = Counter + 1;
    state Anfahrpunkt_5
      entry:
      x_soll = 900;
      y_soll = 800;
    state Wechsel_5
      entry:
      Counter = Counter + 1;
    state Anfahrpunkt_6
      entry:
      x_soll = 600;
      y_soll = 850;
    state Wechsel_6
      entry:
      Counter = Counter + 1;
    state Anfahrpunkt_7
      entry:
      x_soll = 500;
      y_soll = 850;
    state Wechsel_7
      entry:
      Counter = Counter + 1;
    state Anfahrpunkt_8
      entry:
      x_soll = 325;
      y_soll = 800;
    state Wechsel_8
      entry:
      Counter = Counter + 1;
    state Anfahrpunkt_9
      entry:
      x_soll = 240;
      y_soll = 725;
    state Wechsel_9
      entry:
      Counter = Counter + 1;
    state Anfahrpunkt_10
      entry:
      x_soll = 400;
      y_soll = 50;
    state Wechsel_10
      entry:
      Counter = Counter + 1;
    state Anfahrpunkt_11
      entry:
      x_soll = 1200;
      y_soll = 50;
    state Wechsel_11
      entry:
      Counter = Counter + 1;
    state Anfahrpunkt_12
      entry:
      x_soll = 1420;
      y_soll = -100;
    state Wechsel_12
      entry:
      Counter = Counter + 1;
    (default) -> Sammeln.Anfahrpunkt_1 : {Counter = 0}
    Sammeln.Anfahrpunkt_1 -> Sammeln.Wechsel_1 : [abs(x_soll - x_ist) <= Zielradius && abs(y_soll - y_ist) <= Zielradius]
    Sammeln.Wechsel_1 -> Sammeln.Anfahrpunkt_2
    Sammeln.Anfahrpunkt_2 -> Sammeln.Wechsel_2 : [abs(x_soll - x_ist) <= Zielradius && abs(y_soll - y_ist) <= Zielradius]
    Sammeln.Wechsel_2 -> Sammeln.Anfahrpunkt_3
    Sammeln.Anfahrpunkt_3 -> Sammeln.Wechsel_3 : [abs(x_soll - x_ist) <= Zielradius && abs(y_soll - y_ist) <= Zielradius]
    Sammeln.Wechsel_3 -> Sammeln.Anfahrpunkt_4
    Sammeln.Anfahrpunkt_4 -> Sammeln.Wechsel_4 : [abs(x_soll - x_ist) <= Zielradius && abs(y_soll - y_ist) <= Zielradius]
    Sammeln.Wechsel_4 -> Sammeln.Anfahrpunkt_5
    Sammeln.Anfahrpunkt_5 -> Sammeln.Wechsel_5 : [abs(x_soll - x_ist) <= Zielradius && abs(y_soll - y_ist) <= Zielradius]
    Sammeln.Wechsel_5 -> Sammeln.Anfahrpunkt_6
    Sammeln.Anfahrpunkt_6 -> Sammeln.Wechsel_6 : [abs(x_soll - x_ist) <= Zielradius && abs(y_soll - y_ist) <= Zielradius]
    Sammeln.Wechsel_6 -> Sammeln.Anfahrpunkt_7
    Sammeln.Anfahrpunkt_7 -> Sammeln.Wechsel_7 : [abs(x_soll - x_ist) <= Zielradius && abs(y_soll - y_ist) <= Zielradius]
    Sammeln.Wechsel_7 -> Sammeln.Anfahrpunkt_8
    Sammeln.Anfahrpunkt_8 -> Sammeln.Wechsel_8 : [abs(x_soll - x_ist) <= Zielradius && abs(y_soll - y_ist) <= Zielradius]
    Sammeln.Wechsel_8 -> Sammeln.Anfahrpunkt_9
    Sammeln.Anfahrpunkt_9 -> Sammeln.Wechsel_9 : [abs(x_soll - x_ist) <= Zielradius && abs(y_soll - y_ist) <= Zielradius]
    Sammeln.Wechsel_9 -> Sammeln.Anfahrpunkt_10
    Sammeln.Anfahrpunkt_10 -> Sammeln.Wechsel_10 : [abs(x_soll - x_ist) <= Zielradius && abs(y_soll - y_ist) <= Zielradius]
    Sammeln.Wechsel_10 -> Sammeln.Anfahrpunkt_11
    Sammeln.Anfahrpunkt_11 -> Sammeln.Wechsel_11 : [abs(x_soll - x_ist) <= Zielradius && abs(y_soll - y_ist) <= Zielradius]
    Sammeln.Wechsel_11 -> Sammeln.Anfahrpunkt_12
    Sammeln.Anfahrpunkt_12 -> Sammeln.Wechsel_12 : [abs(x_soll - x_ist) <= Zielradius && abs(y_soll - y_ist) <= Zielradius]
  state Schaltung_Gang_Weiterleitung
    Gang = Schaltung;
  state Ende
    entry:
    Gang = 2;
  Sammeln3 -> Uebergabe3 [commented out] : [Counter == 11]
      | {Gang = 1;
      | x_least = x_soll;
      | y_least = y_soll;}
  Uebergabe3 -> Parken3 [commented out] : [Counter == 2]{Gang = 0}
  Sammeln2 -> Uebergabe2 [commented out] : [Counter == 15]
      | {Gang = 1;
      | x_least = x_soll;
      | y_least = y_soll;}
  Uebergabe2 -> Parken2 [commented out] : [Counter == 2]{Gang = 0}
  (default) -> Start_Einstellung_Init
  Sammeln1 -> Uebergabe1 [commented out] : [Counter == 13]
      | {Gang = 1;
      | x_least = x_soll;
      | y_least = y_soll;}
  Uebergabe1 -> Parken1 [commented out] : [Counter == 2]{Gang = 0}
  Start_Einstellung_Init -> (junction 137)
  Sammeln -> Uebergabe : [Counter == 12]
      | {Gang = 1;
      | x_least = x_soll;
      | y_least = y_soll;}
  (junction 137) -> Schaltung_Gang_Weiterleitung [order 2]
  (junction 137) -> Sammeln [order 1] : [Simulation == 1]{Gang = 0}
  Uebergabe -> Parken : [Counter == 2]{Gang = 0}
  Parken -> Ende : [Counter == 3]
  data: x_soll output; y_soll output; Zielradius output; x_ist input; y_ist input; Counter local; x_least local; y_least local; Schaltung input; Simulation input; Gang output

== matlab function Nexonar_Test/Positionsregelungssystem (Soll-Ist-Abgleich & PWM-Auswertung)/PWM-Vektorbetrag ==
  data: pwm_x input; pwm_out output; pwm_y input
function pwm_out = fcn(pwm_x, pwm_y)

pwm_out = round(sqrt(pwm_x * pwm_x + pwm_y * pwm_y));

== stateflow chart Nexonar_Test/Positionsdatengeber [Block "Einstellung_Init" einstellbar] Simulation 1: Fahrsimulation Simulation 2: Datensimulation ==
  state Start_Init_Fahrsimulation
    x_Wagen = Start_x;
    y_Wagen = Start_y;
    alpha_ist = Start_alpha;
    x_ist = x_Wagen + round(r_Versatz_Nexo * cos((phi_Versatz_Nexo+alpha_ist)*2*pi/360));
    y_ist = y_Wagen + round(r_Versatz_Nexo * sin((phi_Versatz_Nexo+alpha_ist)*2*pi/360));
    x_soll = 0;
    y_soll = 0;
  state Fahrsimulation
    state Fahren_mit_Ausrichtungsregelung
      alpha_ist = alpha_ist + Schrittweite(2);
      x_Wagen = x_Wagen + round(Schrittweite(1) * cos(alpha_ist*2*pi/360+pi*Schaltung));
      y_Wagen = y_Wagen + round(Schrittweite(1) * sin(alpha_ist*2*pi/360+pi*Schaltung));
      x_ist = x_Wagen + round(r_Versatz_Nexo * cos((phi_Versatz_Nexo+alpha_ist)*2*pi/360));
      y_ist = y_Wagen + round(r_Versatz_Nexo * sin((phi_Versatz_Nexo+alpha_ist)*2*pi/360));
    state Drehen
      alpha_ist = alpha_ist + Schrittweite(2);
      x_ist = x_Wagen + round(r_Versatz_Nexo * cos((phi_Versatz_Nexo+alpha_ist)*2*pi/360));
      y_ist = y_Wagen + round(r_Versatz_Nexo * sin((phi_Versatz_Nexo+alpha_ist)*2*pi/360));
    (junction 190) -> (junction 192) [order 1] : [alpha_ist + Schrittweite(2) >= 360]
        | {alpha_ist = alpha_ist - 360}
    (junction 192) -> Fahren_mit_Ausrichtungsregelung [order 2]
    Fahren_mit_Ausrichtungsregelung -> (junction 138)
    (junction 190) -> (junction 192) [order 2] : [alpha_ist + Schrittweite(2) < 0]
        | {alpha_ist = alpha_ist + 360}
    (default) -> (junction 190)
    (junction 190) -> (junction 192) [order 3]
    (junction 192) -> Drehen [order 1] : [Schrittweite(1) == 0]
    Drehen -> (junction 138)
    (junction 138) -> (junction 190) : {Schaltung = Gang}
  state Einstellung_Init
    %% Einstellungen allgemein
    Start_x = 1640;
    Start_y = -40;
    Start_alpha = 90 % nur 0 – 359 in Fahrsimulation
    %% Einstellungen für Fahrsimulation
    r_Versatz_Nexo = 10;
    phi_Versatz_Nexo = 195;
    %% Einstellungen für Datensimulation
    Anfang_x = 0;
    Anfang_y = 0;
    Pos_max = 1000;
    Winkel_max = 360;
    Pos_Schritt = 200;   % > 0
    Winkel_Schritt = 20; % > 0
  state Ende
  state Start_Init_Datensimulation
    x_Wagen = 0;
    y_Wagen = 0;
    alpha_ist = Start_alpha;
    x_ist = Start_x;
    y_ist = Start_y;
    x_soll = Anfang_x;
    y_soll = Anfang_y;
  state Datensimulation
    state x_ist_Counter
      x_ist = x_ist + Pos_Schritt;
    state x_soll_Counter
      x_soll = x_soll + Pos_Schritt;
    state alpha_ist_Counter
      alpha_ist = alpha_ist + Winkel_Schritt;
    state y_ist_Counter
      y_ist = y_ist + Pos_Schritt;
    state y_soll_Counter
      y_soll = y_soll + Pos_Schritt;
    state Gangwechsel
      Schaltung = Schaltung + 1;
    (junction 195) -> Gangwechsel [order 2] : [y_ist + Pos_Schritt > Pos_max && x_soll + Pos_Schritt > Pos_max && y_soll + Pos_Schritt > Pos_max && alpha_ist + Winkel_Schritt >= Winkel_max]
        | {x_ist = Start_x; y_ist = Start_y; x_soll = Anfang_x; y_soll = Anfang_y, alpha_ist = Start_alpha;}
    (junction 195) -> alpha_ist_Counter [order 3] : [y_ist + Pos_Schritt > Pos_max && x_soll + Pos_Schritt > Pos_max && y_soll + Pos_Schritt > Pos_max]
        | {x_ist = Start_x; y_ist = Start_y; x_soll = Anfang_x; y_soll = Anfang_y;}
    (default) -> (junction 195)
    (junction 195) -> y_soll_Counter [order 4] : [y_ist + Pos_Schritt > Pos_max && x_soll + Pos_Schritt > Pos_max]
        | {x_ist = Start_x; y_ist = Start_y;
        | x_soll = Anfang_x;}
    Gangwechsel -> (junction 195)
    alpha_ist_Counter -> (junction 195)
    y_soll_Counter -> (junction 195)
    (junction 195) -> x_soll_Counter [order 5] : [y_ist + Pos_Schritt > Pos_max]
        | {x_ist = Start_x;
        | y_ist = Start_y;}
    x_soll_Counter -> (junction 195)
    (junction 195) -> y_ist_Counter [order 6] : {x_ist = Start_x}
    y_ist_Counter -> (junction 195)
    (junction 195) -> x_ist_Counter [order 1] : [x_ist + Pos_Schritt <= Pos_max]
    x_ist_Counter -> (junction 195)
  Fahrsimulation -> Ende : [Schaltung == 2]
  Start_Init_Fahrsimulation -> Fahrsimulation : {Schaltung = Gang}
  (junction 102) -> Start_Init_Fahrsimulation [order 1] : [Simulation == 1]
  Einstellung_Init -> (junction 102)
  (default) -> Einstellung_Init
  (junction 102) -> Start_Init_Datensimulation [order 2]
  Datensimulation -> Ende : [Schaltung == 2]
  Start_Init_Datensimulation -> Datensimulation : {Schaltung = 0}
  data: Gang input double; x_ist output; y_ist output; alpha_ist output; Schaltung output; Pos_max local; Pos_Schritt local; Winkel_Schritt local; Schrittweite input double; Simulation input; Start_x local; Start_y local; Start_alpha local; Anfang_x local; Anfang_y local; Winkel_max local; r_Versatz_Nexo local; phi_Versatz_Nexo local; x_Wagen output; y_Wagen output; x_soll output; y_soll output

== matlab function Nexonar_Test/Schrittweite-Funktionsblock [Init: Fahrgenauigkeit = 10] [Init: Drehgenauigkeit = 30] [Init: Regelgenauigkeit = 2] ==
  data: pwm_out_l input; Schrittweite output; pwm_out_r input; r_l_out_l input; r_l_out_r input
function Schrittweite = fcn(pwm_out_l, pwm_out_r, r_l_out_l, r_l_out_r)

Fahrgenauigkeit = 14; % bis 141
Drehgenauigkeit = 28; % bis 141
Regelgenauigkeit = 1; % bis 10


Schrittweite = [0 0];
if r_l_out_l == r_l_out_r
    Schrittweite(1) = round(sqrt(pwm_out_l * pwm_out_l + pwm_out_r * pwm_out_r) / Fahrgenauigkeit);
    % Fahren Wertebereich brutto: 0 - 141
    Schrittweite(2) = round((pwm_out_r - pwm_out_l) / Regelgenauigkeit) * (1 + (r_l_out_l - 1) * 2);
    % Fahrregelung Wertebereich brutto: 0 - 10
else
    Schrittweite(1) = 0;
    Schrittweite(2) = round(sqrt(pwm_out_l * pwm_out_l + pwm_out_r * pwm_out_r) / Drehgenauigkeit) * (r_l_out_r - r_l_out_l);
    % Drehen Wertebereich brutto: 0 - 141
end

== stateflow chart Nexonar_Test/Fahrsystem ==
  state Fahren_mit_Ausrichtungsregelung
    entry:
    pwm_out_l = pwm_out - round(pwm_mindern(1) * (pwm_out / 100) ^ 2) * l_mindern;
    pwm_out_r = pwm_out - round(pwm_mindern(1) * (pwm_out / 100) ^ 2) * r_mindern;
    r_l_out_l = 1 - Gang;
    r_l_out_r = 1 - Gang;
  state Start_Warten
  state Drehen_links_max
    entry:
    pwm_out_l = 100;
    pwm_out_r = 100;
    r_l_out_l = 0;
    r_l_out_r = 1;
  state Drehen_rechts_max
    entry:
    pwm_out_l = 100;
    pwm_out_r = 100;
    r_l_out_l = 1;
    r_l_out_r = 0;
  state Drehen_links_gesteuert
    entry:
    pwm_out_l = 59 + abs(alpha_diff_opt);
    pwm_out_r = 59 + abs(alpha_diff_opt);
    r_l_out_l = 0;
    r_l_out_r = 1;
  state Drehen_rechts_gesteuert
    entry:
    pwm_out_l = 59 + abs(alpha_diff_opt);
    pwm_out_r = 59 + abs(alpha_diff_opt);
    r_l_out_l = 1;
    r_l_out_r = 0;
  (junction 81) -> Fahren_mit_Ausrichtungsregelung [order 1] : [pwm_mindern(2) == 1]
      | {l_mindern = 1 - Gang; r_mindern = 0 + Gang;}
  (junction 81) -> Fahren_mit_Ausrichtungsregelung [order 2] : [pwm_mindern(2) == 0]
      | {l_mindern = 0 + Gang; r_mindern = 1 - Gang;}
  (junction 1) -> (junction 81) [order 2]
  Fahren_mit_Ausrichtungsregelung -> (junction 32)
  (junction 81) -> Fahren_mit_Ausrichtungsregelung [order 3] : {l_mindern = 0; r_mindern = 0;}
  Start_Warten -> (junction 1)
  (junction 32) -> (junction 1)
  (default) -> Start_Warten
  Drehen_links_max -> (junction 32)
  Drehen_rechts_max -> (junction 32)
  Drehen_links_gesteuert -> (junction 32)
  (junction 1) -> (junction 18) [order 1] : [abs(alpha_diff_opt) > 0 && pwm_out > 0]
  Drehen_rechts_gesteuert -> (junction 32)
  (junction 18) -> (junction 44) [order 1] : [abs(alpha_diff_opt) > 40]
  (junction 44) -> Drehen_links_max [order 1] : [alpha_diff_opt > 0]
  (junction 18) -> (junction 52) [order 2]
  (junction 44) -> Drehen_rechts_max [order 2]
  (junction 52) -> Drehen_links_gesteuert [order 1] : [alpha_diff_opt > 0]
  (junction 52) -> Drehen_rechts_gesteuert [order 2]
  data: Gang input; pwm_out input; pwm_mindern input; alpha_diff_opt input; pwm_out_l output; pwm_out_r output; r_l_out_l output; r_l_out_r output; l_mindern local; r_mindern local

== stateflow chart Nexonar_Test/Drehweg-Optimierung mit Gang-Ausrichtung [Init: Stillstandintervall = ±5°] ==
  state Einstellung_Init
    entry:
    Stillstandintervall = 10;
    %%%
    pwm_mindern = [0 0];
  state Drehstillstand_mit_Ausrichtungsregelung
    entry:
    alpha_diff_opt = 0;
    if abs(alpha_diff_intern) < 5
    pwm_mindern(1) = round(abs(alpha_diff_intern));
    elseif abs(alpha_diff_intern) < 15
    pwm_mindern(1) = 5 + floor((abs(alpha_diff_intern) - 5) / 2);
    else
    pwm_mindern(1) = 10;
    end;
    if alpha_diff_intern < 0
    pwm_mindern(2) = 0;
    elseif alpha_diff_intern > 0
    pwm_mindern(2) = 1;
    else
    pwm_mindern(2) = 2;
    end;
  state Weiterleitung_bei_Drehzustand
    entry:
    alpha_diff_opt = alpha_diff_intern;
  (default) -> Einstellung_Init
  (junction 95) -> (junction 32)
  Einstellung_Init -> (junction 32)
  (junction 32) -> (junction 6) : {alpha_diff_intern = alpha_diff + 180 * Gang}
  (junction 6) -> (junction 68) [order 2]
  (junction 68) -> Drehstillstand_mit_Ausrichtungsregelung [order 1] : [abs(alpha_diff_intern) <= Stillstandintervall]
  Drehstillstand_mit_Ausrichtungsregelung -> (junction 95)
  (junction 6) -> (junction 13) [order 1] : [abs(alpha_diff_intern) > 180]
  (junction 13) -> (junction 68) [order 1] : [alpha_diff_intern > 0]
      | {alpha_diff_intern = -360 + alpha_diff_intern}
  Weiterleitung_bei_Drehzustand -> (junction 95)
  (junction 13) -> (junction 68) [order 2] : {alpha_diff_intern = 360 + alpha_diff_intern}
  (junction 68) -> Weiterleitung_bei_Drehzustand [order 2]
  data: pwm_mindern output; Gang input; alpha_diff input; alpha_diff_opt output; alpha_diff_intern local; Stillstandintervall local

== stateflow chart Nexonar_Test/Winkelregelungssystem (Soll-Ist-Abgleich & Ausrichtungsauswertung)/Quadrantenteiler ==
  state Quadrant_a
    entry:
    Quadrant = 0;
  state Quadrant_b
    entry:
    Quadrant = 1;
  state Start_Warten
  state Quadrant_c
    entry:
    Quadrant = 2;
  state Quadrant_d
    entry:
    Quadrant = 3;
  (junction 6) -> Quadrant_a [order 1] : [x_diff >= 0 && y_diff >= 0]
  Quadrant_a -> (junction 35)
  (junction 6) -> Quadrant_b [order 2] : [x_diff <= 0 && y_diff > 0]
  Quadrant_b -> (junction 35)
  Start_Warten -> (junction 6)
  (junction 35) -> (junction 6)
  (default) -> Start_Warten
  (junction 6) -> Quadrant_c [order 3] : [x_diff < 0 && y_diff <= 0]
  Quadrant_c -> (junction 35)
  (junction 6) -> Quadrant_d [order 4]
  Quadrant_d -> (junction 35)
  data: x_diff input; y_diff input; Quadrant output
